simulink model "chap7_3sim"  (Simulink 8.1)
settings: Solver=ode5  StartTime=0.0  StopTime=10  FixedStep=0.001  RelTol=1e-3
settings Model: Creator=hp  LastModifiedBy=liujk
settings OptimizationCC: InitFltsAndDblsToZero=on
settings DebuggingCC: SaveWithParameterizedLinksMsg=none  SignalResolutionControl=TryResolveAllWithWarning  SolverPrmCheckMsg=none  MultiTaskDSMMsg=warning  MultiTaskCondExecSysMsg=none  StrictBusMsg=Warning
settings RTWCC: IncludeERTFirstTime=on
settings GRTTargetCC: TargetFcnLib=ansi_tfl_tmw.mat

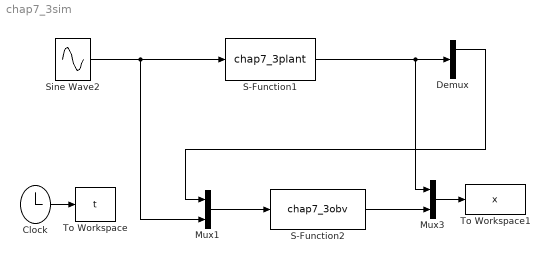
== system chap7_3sim ==
  Clock : Clock
      settings: Decimation=30
  Demux : Demux  Outputs=2
  Mux1 : Mux  Inputs=2
  Mux3 : Mux  Inputs=2
  S-Function1 : S-Function  FunctionName=chap7_3plant  EnableBusSupport=off
  S-Function2 : S-Function  FunctionName=chap7_3obv  EnableBusSupport=off
  Sine Wave2 : Sin  SampleTime=0
  To Workspace : ToWorkspace  VariableName=t  SampleTime=-1
  To Workspace1 : ToWorkspace  VariableName=x  SampleTime=-1
  wires:
  Clock/1 -> To Workspace/1
  Sine Wave2/1 -> S-Function1/1, Mux1/2
  S-Function2/1 -> Mux3/2
  S-Function1/1 -> Demux/1, Mux3/1
  Mux3/1 -> To Workspace1/1
  Demux/1 -> Mux1/1
  Mux1/1 -> S-Function2/1
